simulink subsystem "unity_emitter"  (R2022a)
settings: Solver=VariableStepAuto  StartTime=0.0  StopTime=10.0  RelTol=1e-3
libraries: slrealtimeiplib x1
settings Model: Creator=samuel  LastModifiedBy=samuel

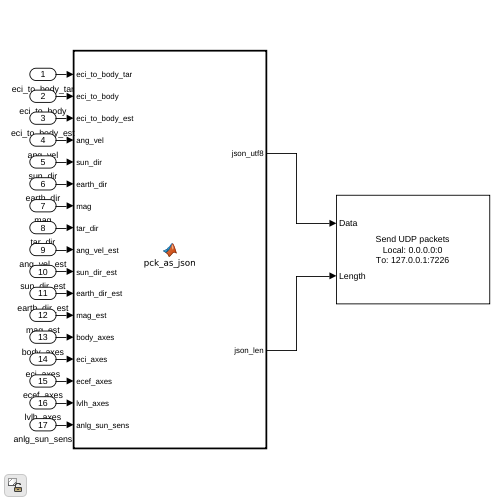
[thumbnail: Simulink's stored preview of the top-level diagram]
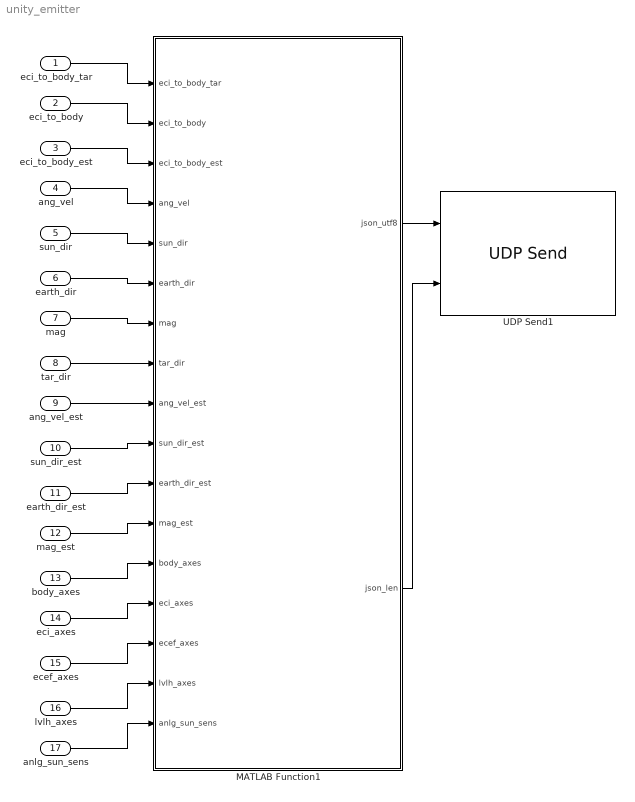
== system unity_emitter ==
  eci_to_body_tar : Inport
  eci_to_body : Inport  Port=2
  eci_to_body_est : Inport  Port=3
  ang_vel : Inport  Port=4
  sun_dir : Inport  Port=5
  earth_dir : Inport  Port=6
  mag : Inport  Port=7
  tar_dir : Inport  Port=8
  ang_vel_est : Inport  Port=9
  sun_dir_est : Inport  Port=10
  earth_dir_est : Inport  Port=11
  mag_est : Inport  Port=12
  body_axes : Inport  Port=13
  eci_axes : Inport  Port=14
  ecef_axes : Inport  Port=15
  lvlh_axes : Inport  Port=16
  anlg_sun_sens : Inport  Port=17
  MATLAB Function1 : MATLAB Function  TreatAsAtomicUnit=on
  UDP Send1 : slrealtimeiplib/UDP Send  useHostTargetConn=off  toAddress=127.0.0.1  toPort=7226  sampleTime=5/60  enableMessage=off
      settings: SourceProductBaseCode=XP
  wires:
  eci_to_body_tar/1 -> MATLAB Function1/1(eci_to_body_tar)
  eci_to_body/1 -> MATLAB Function1/2(eci_to_body)
  anlg_sun_sens/1 -> MATLAB Function1/17(anlg_sun_sens)
  ang_vel_est/1 -> MATLAB Function1/9(ang_vel_est)
  eci_axes/1 -> MATLAB Function1/14(eci_axes)
  tar_dir/1 -> MATLAB Function1/8(tar_dir)
  earth_dir_est/1 -> MATLAB Function1/11(earth_dir_est)
  ecef_axes/1 -> MATLAB Function1/15(ecef_axes)
  MATLAB Function1/1(json_utf8) -> UDP Send1/1
  MATLAB Function1/2(json_len) -> UDP Send1/2
  sun_dir_est/1 -> MATLAB Function1/10(sun_dir_est)
  mag_est/1 -> MATLAB Function1/12(mag_est)
  sun_dir/1 -> MATLAB Function1/5(sun_dir)
  earth_dir/1 -> MATLAB Function1/6(earth_dir)
  eci_to_body_est/1 -> MATLAB Function1/3(eci_to_body_est)
  ang_vel/1 -> MATLAB Function1/4(ang_vel)
  mag/1 -> MATLAB Function1/7(mag)
  lvlh_axes/1 -> MATLAB Function1/16(lvlh_axes)
  body_axes/1 -> MATLAB Function1/13(body_axes)

== matlab function unity_emitter/MATLAB Function1 ==
  data: eci_to_body_tar input size=4; eci_to_body input size=4; eci_to_body_est input size=4; ang_vel input size=3; sun_dir input size=3; earth_dir input size=3; mag input size=3; tar_dir input size=3; ang_vel_est input size=3; sun_dir_est input size=3; earth_dir_est input size=3; mag_est input size=3; json_utf8 output size=1024; json_len output size=1; body_axes input size=9; eci_axes input size=9; ecef_axes input size=9; lvlh_axes input size=9; anlg_sun_sens input size=6
function [json_utf8, json_len] = pck_as_json(eci_to_body_tar, ...
    eci_to_body, eci_to_body_est, ang_vel, sun_dir, ...
    earth_dir, mag, tar_dir, ang_vel_est, sun_dir_est, earth_dir_est, ...
    mag_est, body_axes, eci_axes, ecef_axes, lvlh_axes, anlg_sun_sens)

% initializes the values (needed for initialization)
json_utf8 = uint8(zeros(1024, 1));
json_len = double(0); %#ok This is needed for informing Simulink about size
s = struct;

% Needed to allow jsonencode to be run by the MATLAB engine (as is
% note supported directly through codegen
coder.extrinsic('jsonencode');

% Sets the values in the struct. Note that the single() usage converts the
% value represnetations from double-precision floating point numbers to
% single-precision (given that Unity only uses single-precision)

% Quaternions
s.eci_to_body_tar = single(eci_to_body_tar);
s.eci_to_body = single(eci_to_body);
s.eci_to_body_est = single(eci_to_body_est);

% Vectors
s.ang_vel = ang_vel;
s.sun_dir = sun_dir;
s.earth_dir = earth_dir;
s.mag = mag;
s.tar_dir = tar_dir;

% Estimated vectors
s.ang_vel_est = ang_vel_est;
s.sun_dir_est = sun_dir_est;
s.earth_dir_est = earth_dir_est;
s.mag_est = mag_est;

% Axes
s.body_axes = single(body_axes);
s.eci_axes = single(eci_axes);
s.ecef_axes = single(ecef_axes);
s.lvlh_axes = single(lvlh_axes);

% Sensors
s.anlg_sun_sens = single(anlg_sun_sens);

% Produces the JSON data through serializing the struct
json_str = jsonencode(s);
json_len = strlength(json_str); % Finds the data size

% Moves this new data to the fixed size output in uint8 format
json_utf8(1:json_len) = json_str;
